simulink model "control_model_case_3"  (R2018a)
settings: Solver=VariableStepAuto  StartTime=0.0  StopTime=35  RelTol=1e-3
undefined symbols (not defined in the file): sigbuilder_block
libraries: fuzblock x1
settings Model: Creator=siati  LastModifiedBy=siati

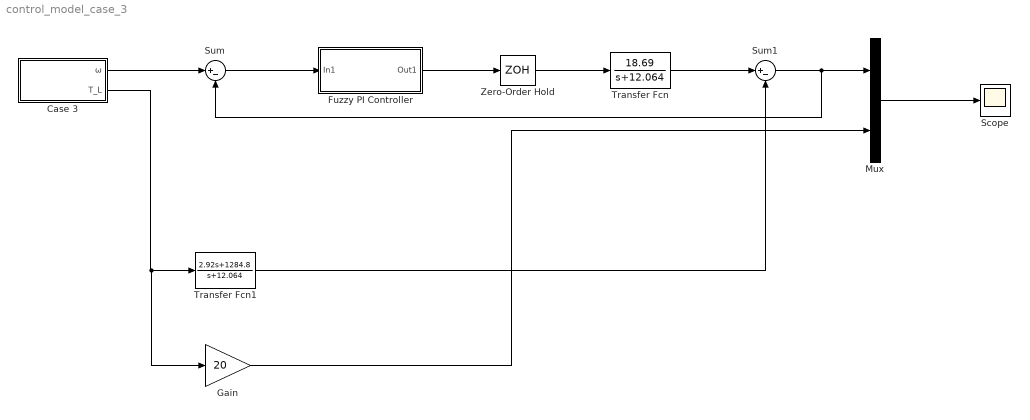
== system control_model_case_3 ==
  Case 3 : Subsystem  Tag=STV Subsys  LoadFcn=sigbuilder_block('load');  StartFcn=sigbuilder_block('start');  StopFcn=sigbuilder_block('stop');  ClipboardFcn=sigbuilder_block('clipboard');  mask(Sigbuilder block){tuvar=[0:10]}
      mask help: Simulink:masks:SigbuilderBlock_MD
      mask init:
      | if ~strcmp(get_param(bdroot(gcbh),'SimulationStatus'),'stopped') tuvar = sigbuilder_block('maskInit'); end
      settings: CopyFcn=sigbuilder_block('copy');  DeleteFcn=sigbuilder_block('delete');  ModelCloseFcn=sigbuilder_block('modelClose');  PreSaveFcn=sigbuilder_block('preSave');  PauseFcn=sigbuilder_block('pause');  ContinueFcn=sigbuilder_block('continue');  NameChangeFcn=sigbuilder_block('namechange');  OpenFcn=sigbuilder_block('open',[627 162.75 550.5 399.75 ]);  CloseFcn=sigbuilder_block('close');
      mask Display: plot(0, 0, 100, 100,[2, 2, 32, 32, 2], [68, 8, 8, 68, 68],[32, 2], [38, 38], [32, 19, 2],[53, 60, 44], [32, 17, 17, 2],[16, 16, 31, 31]);txt = getActiveGroup(gcbh);text(2, 100, txt,'verticalAlignment', 'top');
  Fuzzy PI Controller : Subsystem
  Gain : Gain  Gain=20
  Mux : Mux  Inputs=2
  Scope : Scope
  Sum : Sum  Inputs=|+-
  Sum1 : Sum  Inputs=|+-
  Transfer Fcn : TransferFcn  Numerator=[18.69]  Denominator=[1 12.064]
  Transfer Fcn1 : TransferFcn  Numerator=[2.92 1284.8]  Denominator=[1 12.064]
  Zero-Order Hold : ZeroOrderHold  SampleTime=-1
  wires:
  Sum/1 -> Fuzzy PI Controller/1(In1)
  Fuzzy PI Controller/1(Out1) -> Zero-Order Hold/1
  Zero-Order Hold/1 -> Transfer Fcn/1
  Transfer Fcn/1 -> Sum1/1
  Case 3/1(ω) -> Sum/1
  Case 3/2(T_L) -> Gain/1, Transfer Fcn1/1
  Sum1/1 -> Sum/2, Mux/1
  Transfer Fcn1/1 -> Sum1/2
  Gain/1 -> Mux/2
  Mux/1 -> Scope/1

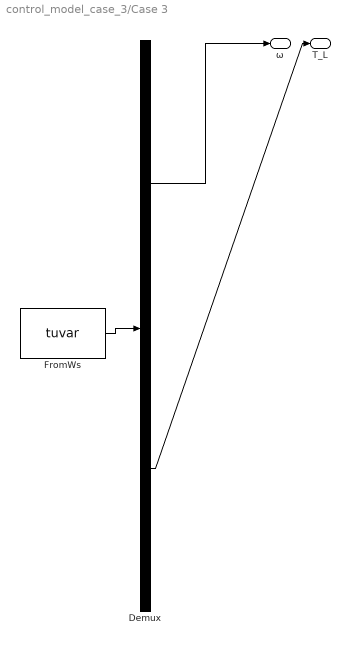
== system control_model_case_3/Case 3 ==
  Demux : Demux  Tag=STV Demux  Outputs=2
  FromWs : FromWorkspace  Tag=STV FromWs  VariableName=tuvar  SampleTime=0
      SigBuilderData=|
      | common.afterFinalStr = 'Extrapolate'
      | common.sampleTime = 0
      | dataSet.timeRange = [0 30]
      | dataSet.name = 'Group 1'
      | sbobj.Groups.Name = 'Group 1'
      | sbobj.Groups.Signals(1).Name = 'ω'
      | sbobj.Groups.Signals(1).XData = [0 30]
      | sbobj.Groups.Signals(1).YData = [150 150]
      | sbobj.Groups.Signals(2).Name = 'T_L'
      | sbobj.Groups.Signals(2).XData = [0 10 10 20 20 30]
      | sbobj.Groups.Signals(2).YData = [0 0 100 100 0 0]
      | sbobj.Groups.TimeRange = [0 30]
  ω : Outport  Tag=STV Outport
  T_L : Outport  Tag=STV Outport  Port=2
  wires:
  Demux/1 -> ω/1
  FromWs/1 -> Demux/1
  Demux/2 -> T_L/1

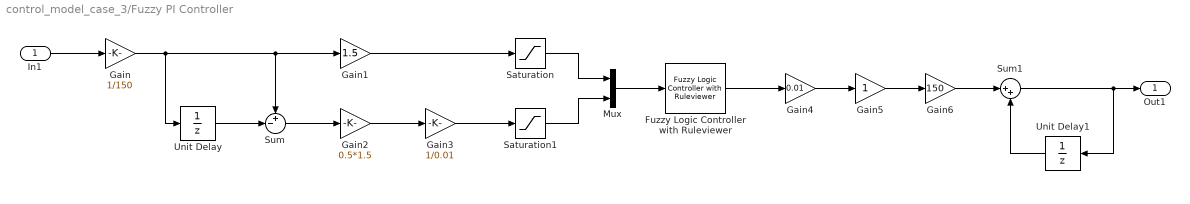
== system control_model_case_3/Fuzzy PI Controller ==
  In1 : Inport
  Fuzzy Logic Controller with Ruleviewer : fuzblock/Fuzzy Logic  Controller  with Ruleviewer  fismatrix=FLC  Ts=1
  Gain : Gain  Gain=1/150
  Gain1 : Gain  Gain=1.5
  Gain2 : Gain  Gain=0.5*1.5
  Gain3 : Gain  Gain=1/0.01
  Gain4 : Gain  Gain=0.01
  Gain5 : Gain
  Gain6 : Gain  Gain=150
  Mux : Mux  Inputs=2
  Saturation : Saturate
  Saturation1 : Saturate
  Sum : Sum  Inputs=+-|
  Sum1 : Sum  Inputs=|++
  Unit Delay : UnitDelay  SampleTime=-1
  Unit Delay1 : UnitDelay  SampleTime=-1
  Out1 : Outport
  wires:
  Gain4/1 -> Gain5/1
  Gain5/1 -> Gain6/1
  In1/1 -> Gain/1
  Gain/1 -> Sum/1, Gain1/1, Unit Delay/1
  Unit Delay/1 -> Sum/2
  Sum/1 -> Gain2/1
  Gain2/1 -> Gain3/1
  Gain1/1 -> Saturation/1
  Gain3/1 -> Saturation1/1
  Saturation/1 -> Mux/1
  Saturation1/1 -> Mux/2
  Mux/1 -> Fuzzy Logic Controller with Ruleviewer/1
  Gain6/1 -> Sum1/1
  Unit Delay1/1 -> Sum1/2
  Sum1/1 -> Out1/1, Unit Delay1/1
  Fuzzy Logic Controller with Ruleviewer/1 -> Gain4/1
